simulink model "Lorenz_final_2020a"  (R2020a)
settings: Solver=VariableStepAuto  StartTime=0.0  StopTime=1000  RelTol=1e-3
model workspace (MAT data in the model file):
  a = 0.001
  b = 0.9
  c = 0.03
settings Model: Creator=RaviM  LastModifiedBy=RaviM
settings DebuggingCC: SFMachineParentedDataDiag=error

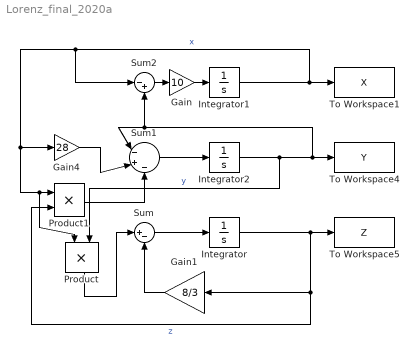
== system Lorenz_final_2020a ==
  Gain : Gain  Gain=10
  Gain1 : Gain  Gain=8/3
  Gain4 : Gain  Gain=28
  Integrator : Integrator  InitialCondition=30
  Integrator1 : Integrator
  Integrator2 : Integrator  InitialCondition=1
  Product : Product
  Product1 : Product
  Sum : Sum  Inputs=|+-
  Sum1 : Sum  Inputs=|-+-
  Sum2 : Sum  Inputs=|-+
  To Workspace1 : ToWorkspace  VariableName=X  SaveFormat=Timeseries  SampleTime=-1
  To Workspace4 : ToWorkspace  VariableName=Y  SaveFormat=Timeseries  SampleTime=-1
  To Workspace5 : ToWorkspace  VariableName=Z  SaveFormat=Timeseries  SampleTime=-1
  wires:
  Integrator1/1 -> Product1/1, Product/1, Gain4/1, Sum2/1, To Workspace1/1  "x"
  Integrator/1 -> Product1/2, Gain1/1, To Workspace5/1  "z"
  Integrator2/1 -> Product/2, To Workspace4/1, Sum1/1, Sum2/2  "y"
  Gain4/1 -> Sum1/2
  Product1/1 -> Sum1/3
  Sum1/1 -> Integrator2/1
  Gain1/1 -> Sum/2
  Sum/1 -> Integrator/1
  Sum2/1 -> Gain/1
  Gain/1 -> Integrator1/1
  Product/1 -> Sum/1
